simulink model "Esercizio2_4"  (R2015b)
settings: Solver=VariableStepAuto  StartTime=0.0  StopTime=500.0  RelTol=1e-3
libraries: fuzblock x5, simulink x3
settings Model: Creator=Cristian  LastModifiedBy=Cristian

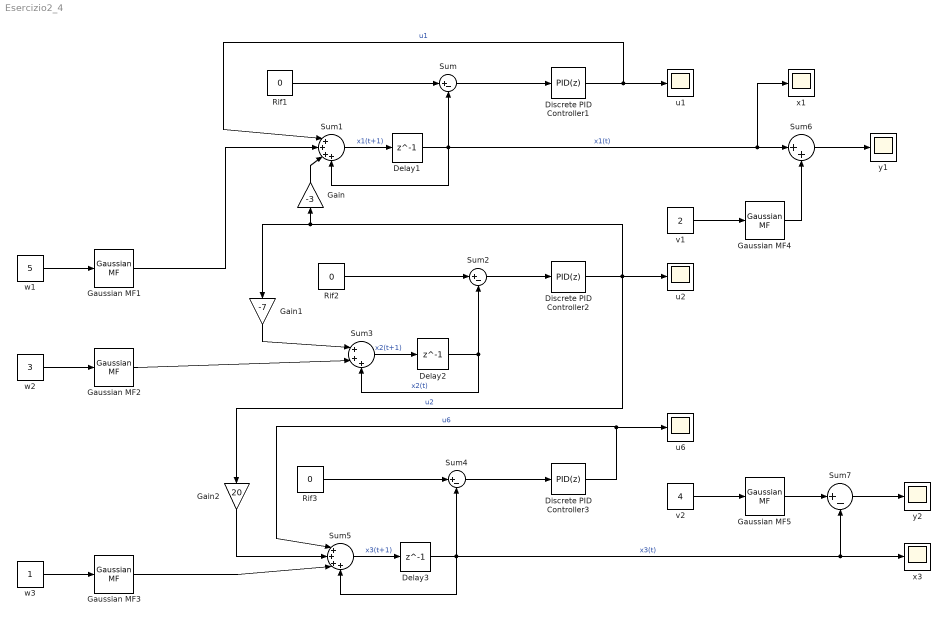
== system Esercizio2_4 ==
  Delay1 : Delay  DelayLength=1  InitialCondition=3
  Delay2 : Delay  DelayLength=1  InitialCondition=5
  Delay3 : Delay  DelayLength=1  InitialCondition=7
  Discrete PID Controller1 : simulink/Continuous/PID Controller  Controller=PID  TimeDomain=Discrete-time  SampleTime=1  IntegratorMethod=Forward Euler  FilterMethod=Forward Euler  Form=Parallel  UseFilter=on  ControllerParametersSource=internal  P=0.02881  I=0.0001535  D=-0.2003  N=0.04707  InitialConditionSource=internal  InitialConditionForIntegrator=0  InitialConditionForFilter=0  ExternalReset=none  LimitOutput=off  UpperSaturationLimit=inf  LowerSaturationLimit=-inf  LinearizeAsGain=off  AntiWindupMode=none  Kb=1  TrackingMode=off  Kt=1  PParamMin=[]  PParamMax=[]  IParamMin=[]  IParamMax=[]  DParamMin=[]  DParamMax=[]  NParamMin=[]  NParamMax=[]  KbParamMin=[]  KbParamMax=[]  KtParamMin=[]  KtParamMax=[]  POutMin=[]  POutMax=[]  IOutMin=[]  IOutMax=[]  DOutMin=[]  DOutMax=[]  NOutMin=[]  NOutMax=[]  KbOutMin=[]  KbOutMax=[]  KtOutMin=[]  KtOutMax=[]  IntegratorOutMin=[]  IntegratorOutMax=[]  FilterOutMin=[]  FilterOutMax=[]  SumOutMin=[]  SumOutMax=[]  SumI1OutMin=[]  SumI1OutMax=[]  SumI2OutMin=[]  SumI2OutMax=[]  SumI3OutMin=[]  SumI3OutMax=[]  SumDOutMin=[]  SumDOutMax=[]  SaturationOutMin=[]  SaturationOutMax=[]  IntegratorContinuousStateAttributes=''  IntegratorStateMustResolveToSignalObject=off  IntegratorRTWStateStorageClass=Auto  FilterContinuousStateAttributes=''  FilterStateMustResolveToSignalObject=off  FilterRTWStateStorageClass=Auto  DifferentiatorICPrevScaledInput=0  DifferentiatorOutMin=[]  DifferentiatorOutMax=[]
  Discrete PID Controller2 : simulink/Continuous/PID Controller  Controller=PID  TimeDomain=Discrete-time  SampleTime=1  IntegratorMethod=Forward Euler  FilterMethod=Forward Euler  Form=Parallel  UseFilter=on  ControllerParametersSource=internal  P=-0.003601  I=-1.9191e-05  D=0.02504  N=0.04707  InitialConditionSource=internal  InitialConditionForIntegrator=0  InitialConditionForFilter=0  ExternalReset=none  LimitOutput=off  UpperSaturationLimit=inf  LowerSaturationLimit=-inf  LinearizeAsGain=off  AntiWindupMode=none  Kb=1  TrackingMode=off  Kt=1  PParamMin=[]  PParamMax=[]  IParamMin=[]  IParamMax=[]  DParamMin=[]  DParamMax=[]  NParamMin=[]  NParamMax=[]  KbParamMin=[]  KbParamMax=[]  KtParamMin=[]  KtParamMax=[]  POutMin=[]  POutMax=[]  IOutMin=[]  IOutMax=[]  DOutMin=[]  DOutMax=[]  NOutMin=[]  NOutMax=[]  KbOutMin=[]  KbOutMax=[]  KtOutMin=[]  KtOutMax=[]  IntegratorOutMin=[]  IntegratorOutMax=[]  FilterOutMin=[]  FilterOutMax=[]  SumOutMin=[]  SumOutMax=[]  SumI1OutMin=[]  SumI1OutMax=[]  SumI2OutMin=[]  SumI2OutMax=[]  SumI3OutMin=[]  SumI3OutMax=[]  SumDOutMin=[]  SumDOutMax=[]  SaturationOutMin=[]  SaturationOutMax=[]  IntegratorContinuousStateAttributes=''  IntegratorStateMustResolveToSignalObject=off  IntegratorRTWStateStorageClass=Auto  FilterContinuousStateAttributes=''  FilterStateMustResolveToSignalObject=off  FilterRTWStateStorageClass=Auto  DifferentiatorICPrevScaledInput=0  DifferentiatorOutMin=[]  DifferentiatorOutMax=[]
  Discrete PID Controller3 : simulink/Continuous/PID Controller  Controller=PID  TimeDomain=Discrete-time  SampleTime=1  IntegratorMethod=Forward Euler  FilterMethod=Forward Euler  Form=Parallel  UseFilter=on  ControllerParametersSource=internal  P=0.02881  I=0.0001535  D=-0.2003  N=0.04707  InitialConditionSource=internal  InitialConditionForIntegrator=0  InitialConditionForFilter=0  ExternalReset=none  LimitOutput=off  UpperSaturationLimit=inf  LowerSaturationLimit=-inf  LinearizeAsGain=off  AntiWindupMode=none  Kb=1  TrackingMode=off  Kt=1  PParamMin=[]  PParamMax=[]  IParamMin=[]  IParamMax=[]  DParamMin=[]  DParamMax=[]  NParamMin=[]  NParamMax=[]  KbParamMin=[]  KbParamMax=[]  KtParamMin=[]  KtParamMax=[]  POutMin=[]  POutMax=[]  IOutMin=[]  IOutMax=[]  DOutMin=[]  DOutMax=[]  NOutMin=[]  NOutMax=[]  KbOutMin=[]  KbOutMax=[]  KtOutMin=[]  KtOutMax=[]  IntegratorOutMin=[]  IntegratorOutMax=[]  FilterOutMin=[]  FilterOutMax=[]  SumOutMin=[]  SumOutMax=[]  SumI1OutMin=[]  SumI1OutMax=[]  SumI2OutMin=[]  SumI2OutMax=[]  SumI3OutMin=[]  SumI3OutMax=[]  SumDOutMin=[]  SumDOutMax=[]  SaturationOutMin=[]  SaturationOutMax=[]  IntegratorContinuousStateAttributes=''  IntegratorStateMustResolveToSignalObject=off  IntegratorRTWStateStorageClass=Auto  FilterContinuousStateAttributes=''  FilterStateMustResolveToSignalObject=off  FilterRTWStateStorageClass=Auto  DifferentiatorICPrevScaledInput=0  DifferentiatorOutMin=[]  DifferentiatorOutMax=[]
  Gain : Gain  Gain=-3
  Gain1 : Gain  Gain=-7
  Gain2 : Gain  Gain=20
  Gaussian MF{1..5} (5 alike) : fuzblock/Membership  Functions/Gaussian MF  sigma=1  mu=0
  Rif1 : Constant  Description=W  Value=0
  Rif2 : Constant  Description=W  Value=0
  Rif3 : Constant  Description=W  Value=0
  Sum{,2,4,7} (4 alike) : Sum  Inputs=|+-
  Sum1 : Sum  Inputs=|++++
  Sum3 : Sum  Inputs=|+++
  Sum5 : Sum  Inputs=|++++
  Sum6 : Sum  Inputs=|++
  u1 : Scope
  u2 : Scope
  u6 : Scope
  v1 : Constant  Description=W  Value=2
  v2 : Constant  Description=W  Value=4
  w1 : Constant  Description=W  Value=5
  w2 : Constant  Description=W  Value=3
  w3 : Constant  Description=W
  x1 : Scope
  x3 : Scope
  y1 : Scope
  y2 : Scope
  wires:
  w1/1 -> Gaussian MF1/1
  Rif1/1 -> Sum/1
  Sum/1 -> Discrete PID Controller1/1
  Delay1/1 -> Sum/2, x1/1, Sum6/1, Sum1/4  "x1(t)"
  Sum1/1 -> Delay1/1  "x1(t+1)"
  Discrete PID Controller1/1 -> Sum1/1, u1/1  "u1"
  w2/1 -> Gaussian MF2/1
  w3/1 -> Gaussian MF3/1
  Gaussian MF1/1 -> Sum1/2
  Rif2/1 -> Sum2/1
  Sum2/1 -> Discrete PID Controller2/1
  Delay2/1 -> Sum3/3, Sum2/2  "x2(t)"
  Sum3/1 -> Delay2/1  "x2(t+1)"
  Discrete PID Controller2/1 -> u2/1, Gain2/1, Gain1/1, Gain/1  "u2"
  Gaussian MF2/1 -> Sum3/2
  Gain/1 -> Sum1/3
  Gain1/1 -> Sum3/1
  Rif3/1 -> Sum4/1
  Sum4/1 -> Discrete PID Controller3/1
  Delay3/1 -> Sum7/2, x3/1, Sum4/2, Sum5/4  "x3(t)"
  Sum5/1 -> Delay3/1  "x3(t+1)"
  Discrete PID Controller3/1 -> Sum5/1, u6/1  "u6"
  Gain2/1 -> Sum5/2
  Gaussian MF3/1 -> Sum5/3
  v1/1 -> Gaussian MF4/1
  v2/1 -> Gaussian MF5/1
  Gaussian MF4/1 -> Sum6/2
  Sum6/1 -> y1/1
  Sum7/1 -> y2/1
  Gaussian MF5/1 -> Sum7/1
